simulink model "RS_DS_CM11_SimulinkRS"  (R2021b)
settings: Solver=ode1  StartTime=0.0  StopTime=Inf  FixedStep=0.001  RelTol=1e-3  EnableMultiTasking=on
PreLoadFcn:
  | if ~length(which('cmcmd')), cmenv; end
PostLoadFcn:
  | if any(exist('dsrtsu_mdlpostloadfcn', 'file') ~= 0), dsrtsu_mdlpostloadfcn('Execute', bdroot); end
InitFcn:
  | , if any(exist('rtifpga_mdlclblib', 'file') ~= 0), rtifpga_mdlclblib('Init', bdroot); end,
  | , if any(exist('dsmpb_private', 'file') ~= 0), dsmpb_private('dsmpb_mdlclblib', 'Init', bdroot); end,
  | runRS_SimulinkRS
values from neighbouring files (symbols this model uses):
  RealSimPara = struct    [runRS_SimulinkRS.m]    (also in runRS_noSimulinkRS.m)
libraries: CarMaker4SL x26, simulink x8, dsmpblib x7
(part 1 of 3)
PreSaveFcn:
  | , if any(exist('dsmpb_private', 'file') ~= 0), dsmpb_private('dsmpb_mdlclblib', 'PreSave', bdroot); end,
CloseFcn:
  | , if any(exist('dsmpb_private', 'file') ~= 0), dsmpb_private('dsmpb_mdlclblib', 'Close', bdroot); end,
settings Model: DSMPB_ID_DATA={'3029',struct('BlockId','959bbced-12c1-4767-83a1-89929a5713b7','SignalIds',{{'2dfba762-4a5d-4fb2-87c1-b3b2aa88a040'}}),'3030',struct('BlockId','c64a001f-194b-4229-bcb5-f85e1cedc51d','SignalIds',{{'b08fdf9a-de67-414c-8e8c-71615b990809'}}),'3031',struct('BlockId','a9d3bfec-9c38-4599-8c4c-82c07529655a','SignalIds',{{'89e99f5d-9eaf-4b55-ad87-136358e30858','260a6fdd-0a39-4666-a4ad-b2eb1261597d'}}),'3032',struct('BlockId','5c03b8fd-28bb-4541-b179-8665d7eb2a0a','SignalIds',{{'517e5a36-3f43-4f7c-bb45-a47e2302358f','00b36bbc-8fea-4739-bdae-9e60071a5ae6','c6bc667d-2809-40ad-8f52-15d7a7d0c444','b5810d90-0e08-4e08-a893-fc1e5645df05'}}),'3033',struct('BlockId','a9f3426c-e708-4ce6-abaa-842916ca8f03','SignalIds',{{'50966301-89aa-49cd-9e83-22a02fa0d1d9'}}),'3034',struct('BlockId','c86d215d-d6c6-481a-aa0d-d548a059715d','SignalIds',{{'abefa9c2-5971-43e2-92ea-8b98002a54ba','cddb9d5a-43dc-4246-b7b3-04f9827e0c24'}}),'3035',struct('BlockId','41a219ac-5dcc-4ef2-a113-31c003cb4a29','SignalIds',{{'3a4e41e0-0059-4009-8606-30e05f8817b4'}})}  RTICANMMDATA=struct('GeneralSetupData',struct('modelroot','C:\CM_Projects\RealSimCm11Prj\src_cm4sl','generalsettings',struct('filesettings',struct('destfolder',struct('Name','RTICANMM_FILES','Check',1),'buildfolder',struct('Name','.','Check',1),'AbsDestfolder',struct('Name','C:\CM_Projects\RealSimCm11Prj\src_cm4sl\RTICANMM_FILES'),'AbsBuildfolder',struct('Name','C:\CM_Projects\RealSimCm11Prj\src_cm4sl'))),'options',struct('addpaths',1,'rmpaths',1,'addtrcexclusion',true,'cannavigator',struct('checkmonitoring',0),'show_usrtrc',0,'use_usrtrc',0),'advanced',struct('options',ones(1,100)),'MPSetup',{{}},'RTI',struct('Type','DSRT','Ver','4.6','Date','02-Nov-2021'),'modelname','RS_DS_CM11_SimulinkRS','block','RS_DS_CM11_SimulinkRS'))  DSRTSU_INTERNAL_RTIFPGA=170  DSRTSU_INTERNAL_RTISTBM_VER=1.4.3  Creator=fh  LastModifiedBy=y0n
settings SolverCC: AlgebraicLoopSolver=TrustRegion
settings DataIOCC: LimitDataPoints=on  SaveFormat=Array  SignalLoggingSaveFormat=ModelDataLogs  ReturnWorkspaceOutputs=off  SignalLoggingName=sigsOut
settings OptimizationCC: BlockReduction=off  BooleanDataType=off  ConditionallyExecuteInputs=off  OptimizeBlockIOStorage=off  BufferReuse=off  GlobalBufferReuse=off  ExpressionFolding=off  ExpressionDepthLimit=2147483647  LocalBlockOutputs=off  InitFltsAndDblsToZero=on  OptimizeDataStoreBuffers=off  BusAssignmentInplaceUpdate=off
settings DebuggingCC: SaveWithParameterizedLinksMsg=none  UnderspecifiedInitializationDetection=Classic  MergeDetectMultiDrivingBlocksExec=none  SignalResolutionControl=TryResolveAllWithWarning  MultiTaskDSMMsg=warning  MultiTaskCondExecSysMsg=none  TasksWithSamePriorityMsg=none  FcnCallInpInsideContextMsg=warning  StateNameClashWarn=warning  SFUnexpectedBacktrackingDiag=warning  SFNoUnconditionalDefaultTransitionDiag=warning  SFMachineParentedDataDiag=warning  ArithmeticOperatorsInVariantConditions=warning
settings HardwareCC: ProdBitPerPointer=32  ProdBitPerSizeT=32  ProdBitPerPtrDiffT=32  ProdLargestAtomicInteger=Integer  ProdWordSize=32  ProdHWDeviceType=Custom Processor->Custom
settings ModelReferenceCC: PropagateSignalLabelsOutOfModel=off
settings SFSimCC: SimUseLocalCustomCode=off  MATLABDynamicMemAlloc=off  CustomCodeUndefinedFunction=UseInterfaceOnly
settings RTWCC: Description=dSPACE Run-Time Target (for VEOS on Windows and ConfigurationDesk)  SystemTargetFile=dsrt.tlc  GenCodeOnly=on  MakeCommand=make_dsrt  TemplateMakefile=dsrt_default_tmf  RTWVerbose=off  RTWUseLocalCustomCode=off
settings CodeAppCC: MaxIdLength=63  StateflowObjectComments=on
settings STFCustomTargetCC: ParMdlRefBuildCompliant=on  GRTInterface=off  SystemTargetFile=dsrt.tlc
settings GRTTargetCC: TargetLangStandard=C89/C90 (ANSI)  CompOptLevelCompliant=off  ConcurrentExecutionCompliant=off  CombineOutputUpdateFcns=off  MatFileLogging=off  CPPClassGenCompliant=off  UseToolchainInfoCompliant=off
settings ConfigComp: CovMetricSettings=dw  CovSaveCumulativeToWorkspaceVar=on  CovSaveSingleToWorkspaceVar=on  CovExternalEMLEnable=off

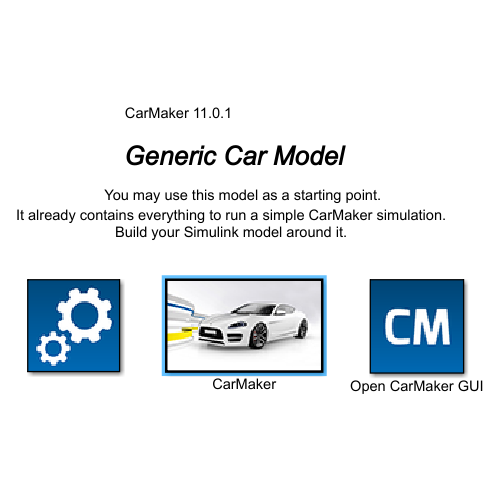
[thumbnail: Simulink's stored preview of the top-level diagram]
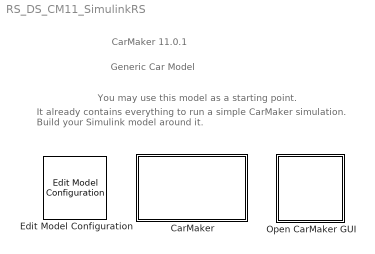
== system RS_DS_CM11_SimulinkRS ==
  note: Generic Car Model
  note: You may use this model as a starting point.
  note: It already contains everything to run a simple CarMaker simulation.
      | Build your Simulink model around it.
  note: CarMaker 11.0.1
  CarMaker : Subsystem  TreatAsAtomicUnit=on
      mask Display: image(imread('CarMakerSys.png'));
  Edit Model Configuration : CarMaker4SL/Edit Model Configuration  SFunctionModules=''
  Open CarMaker GUI : Subsystem  LoadFcn=if ~length(which('cmself')), cmenv; end
      settings: OpenFcn=cmblockmagic('gui_fix_display'); CM_HIL
      mask Display: image(imread('CarMakerGUI.png'));

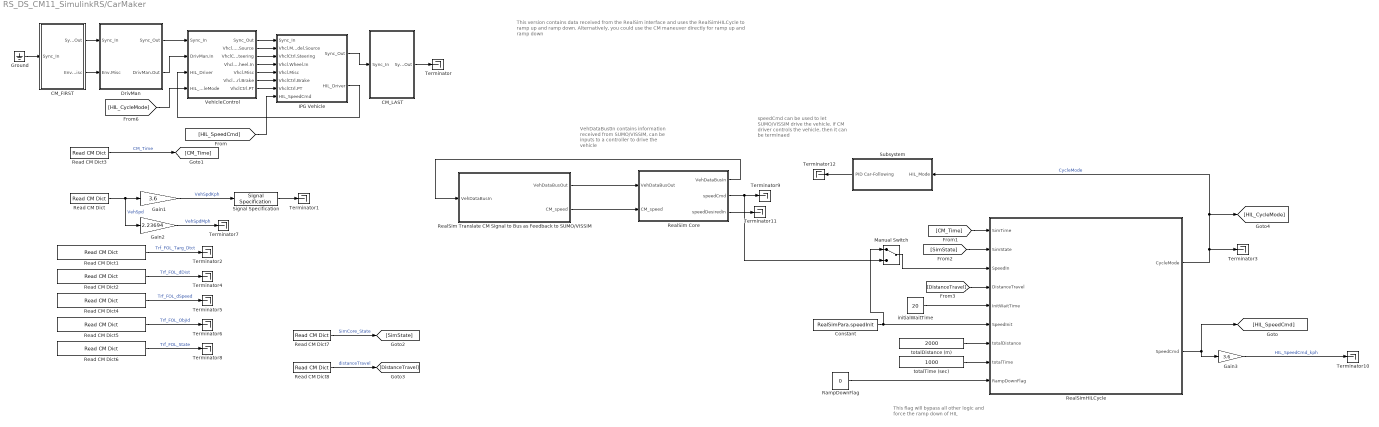
== system RS_DS_CM11_SimulinkRS/CarMaker ==
  note: This version contains data received from the RealSim interface and uses the RealSimHILCycle to ramp up and ramp down.
      |
      | Alternatively, you could use the CM maneuver directly for ramp up and ramp down
  note: speedCmd can be used to let SUMO/VISSIM drive the vehicle. if CM driver controls the vehicle, then it can be terminaed
  note: VehDataBustIn contains information received from SUMO/VISSIM, can be inputs to a controller to drive the vehicle
  note: This flag will bypass all other logic and force the ramp down of HIL
  CM_FIRST : Subsystem
  CM_LAST : Subsystem
  Constant : Constant  Value=RealSimPara.speedInit
  DrivMan : Subsystem
  Gain1 : Gain  Gain=3.6
  Gain2 : Gain  Gain=2.23694
  Gain3 : Gain  Gain=3.6
  Ground : Ground
  IPG Vehicle : Subsystem
  Manual Switch : ManualSwitch
  RampDownFlag : Constant  Value=0
  Read CM Dict : CarMaker4SL/Read CM Dict  xname=Car.v  xsync=off  xstime=Continuous
  Read CM Dict1 : CarMaker4SL/Read CM Dict  xname=Driver.ReCon.Trf_FOL.Targ_Dtct  xsync=off  xstime=Continuous
  Read CM Dict2 : CarMaker4SL/Read CM Dict  xname=Driver.ReCon.Trf_FOL.dDist  xsync=off  xstime=Continuous
  Read CM Dict3 : CarMaker4SL/Read CM Dict  xname=Time  xsync=off  xstime=Continuous
  Read CM Dict4 : CarMaker4SL/Read CM Dict  xname=Driver.ReCon.Trf_FOL.dSpeed  xsync=off  xstime=Continuous
  Read CM Dict5 : CarMaker4SL/Read CM Dict  xname=Driver.ReCon.Trf_FOL.ObjId  xsync=off  xstime=Continuous
  Read CM Dict6 : CarMaker4SL/Read CM Dict  xname=Driver.ReCon.Trf_FOL.State  xsync=off  xstime=Continuous
  Read CM Dict7 : CarMaker4SL/Read CM Dict  xname=SC.State  xsync=off  xstime=Continuous
  Read CM Dict8 : CarMaker4SL/Read CM Dict  xname=Vhcl.Distance  xsync=off  xstime=Continuous
  RealSim Core : Subsystem
  RealSim Translate CM Signal to Bus as Feedback to SUMO/VISSIM : Subsystem
  RealSimHILCycle : Stateflow chart  TreatAsAtomicUnit=on
  Signal Specification : SignalSpecification  Unit=km/h
  Subsystem : Subsystem
  Terminator{,1..12} (13 alike) : Terminator
  VehicleControl : Subsystem
  initialWaitTime : Constant  Value=20
  totalDistance (m) : Constant  Value=2000
  totalTime (sec) : Constant  Value=1000
  wires:
  DrivMan/2(DrivMan.Out) -> VehicleControl/2(DrivMan.In)
  DrivMan/1(Sync_Out) -> VehicleControl/1(Sync_In)
  CM_FIRST/2(Env.Misc) -> DrivMan/2(Env.Misc)
  CM_FIRST/1(Sync_Out) -> DrivMan/1(Sync_In)
  CM_LAST/1(Sync_Out) -> Terminator/1
  Ground/1 -> CM_FIRST/1(Sync_In)
  IPG Vehicle/1(Sync_Out) -> CM_LAST/1(Sync_In)
  VehicleControl/1(Sync_Out) -> IPG Vehicle/1(Sync_In)
  VehicleControl/3(VhclCtrl.Steering) -> IPG Vehicle/3(VhclCtrl.Steering)
  VehicleControl/4(Vhcl.Wheel.In) -> IPG Vehicle/4(Vhcl.Wheel.In)
  VehicleControl/5(Vhcl.Misc) -> IPG Vehicle/5(Vhcl.Misc)
  VehicleControl/6(VhclCtrl.Brake) -> IPG Vehicle/6(VhclCtrl.Brake)
  VehicleControl/7(VhclCtrl.PT) -> IPG Vehicle/7(VhclCtrl.PT)
  VehicleControl/2(Vhcl.Model.Source) -> IPG Vehicle/2(Vhcl.Model.Source)
  Read CM Dict3/1 -> [CM_Time]  "CM_Time"
  Read CM Dict/1 -> Gain2/1, Gain1/1  "VehSpd"
  Gain2/1 -> Terminator7/1  "VehSpdMph"
  Gain1/1 -> Signal Specification/1  "VehSpdKph"
  Signal Specification/1 -> Terminator1/1
  Read CM Dict1/1 -> Terminator2/1  "Trf_FOL_Targ_Dtct"
  Read CM Dict2/1 -> Terminator4/1  "Trf_FOL_dDist"
  Read CM Dict4/1 -> Terminator5/1  "Trf_FOL_dSpeed"
  Read CM Dict5/1 -> Terminator6/1  "Trf_FOL_ObjId"
  Read CM Dict6/1 -> Terminator8/1  "Trf_FOL_State"
  RealSim Core/2(speedCmd) -> Terminator9/1, Manual Switch/2
  RealSim Translate CM Signal to Bus as Feedback to SUMO/VISSIM/2(CM_speed) -> RealSim Core/2(CM_speed)
  RealSim Core/1(VehDataBusIn) -> RealSim Translate CM Signal to Bus as Feedback to SUMO/VISSIM/1(VehDataBusIn)
  RealSim Translate CM Signal to Bus as Feedback to SUMO/VISSIM/1(VehDataBusOut) -> RealSim Core/1(VehDataBusOut)
  Read CM Dict7/1 -> [SimState]  "SimCore_State"
  IPG Vehicle/2(HIL_Driver) -> VehicleControl/3(HIL_Driver)
  RealSim Core/3(speedDesiredIn) -> Terminator11/1
  [HIL_SpeedCmd] -> IPG Vehicle/8(HIL_SpeedCmd)
  Read CM Dict8/1 -> [DistanceTravel]  "distanceTravel"
  [SimState] -> RealSimHILCycle/2(SimState)
  Constant/1 -> RealSimHILCycle/6(SpeedInit), Manual Switch/1
  totalDistance (m)/1 -> RealSimHILCycle/7(totalDistance)
  [DistanceTravel] -> RealSimHILCycle/4(DistanceTravel)
  RealSimHILCycle/2(SpeedCmd) -> [HIL_SpeedCmd], Gain3/1
  Subsystem/1(PID Car-Following) -> Terminator12/1
  initialWaitTime/1 -> RealSimHILCycle/5(InitWaitTime)
  [CM_Time] -> RealSimHILCycle/1(SimTime)
  RealSimHILCycle/1(CycleMode) -> [HIL_CycleMode], Subsystem/1(HIL_Mode), Terminator3/1  "CycleMode"
  totalTime (sec)/1 -> RealSimHILCycle/8(totalTime)
  Manual Switch/1 -> RealSimHILCycle/3(SpeedIn)
  Gain3/1 -> Terminator10/1  "HIL_SpeedCmd_kph"
  RampDownFlag/1 -> RealSimHILCycle/9(RampDownFlag)
  [HIL_CycleMode] -> VehicleControl/4(HIL_CycleMode)

== system RS_DS_CM11_SimulinkRS/Open CarMaker GUI ==
  S-Function : S-Function  FunctionName=cm_gui  SFunctionDeploymentMode=off  EnableBusSupport=off

== system RS_DS_CM11_SimulinkRS/CarMaker/CM_FIRST ==
  Sync_In : Inport
  BusCreator1 : BusCreator  Inputs=8
  BusCreator2 : BusCreator  Inputs=6
  Demux1 : Demux  Outputs=14
      settings: DisplayOption=none
  Environment : S-Function  FunctionName=CM_Sfun  Parameters='Environment'  SFunctionDeploymentMode=off  EnableBusSupport=off
  IoIn : S-Function  FunctionName=CM_Sfun  Parameters='IoIn'  SFunctionDeploymentMode=off  EnableBusSupport=off
  Terminator : Terminator
  Sync_Out : Outport  VectorParamsAs1DForOutWhenUnconnected=off
  Env.Misc : Outport  Port=2  VectorParamsAs1DForOutWhenUnconnected=off
  wires:
  BusCreator2/1 -> Terminator/1  "IF Environment (in)"
  BusCreator1/1 -> Env.Misc/1
  Demux1/14 -> BusCreator2/6  "Env sRoad"
  Demux1/13 -> BusCreator2/5  "Env PoI_GCS Elev"
  Demux1/12 -> BusCreator2/4  "Env PoI_GCS Lat"
  Demux1/11 -> BusCreator2/3  "Env PoI_GCS Long"
  Demux1/10 -> BusCreator2/2  "Env Time"
  Demux1/9 -> BusCreator2/1  "Env yDay"
  Demux1/8 -> BusCreator1/8  "Env WindVel_tot z"
  Demux1/7 -> BusCreator1/7  "Env WindVel_tot y"
  Demux1/6 -> BusCreator1/6  "Env WindVel_tot x"
  Demux1/5 -> BusCreator1/5  "Env SolarRadiation"
  Demux1/4 -> BusCreator1/4  "Env AirHumidity"
  Demux1/3 -> BusCreator1/3  "Env AirPressure"
  Demux1/2 -> BusCreator1/2  "Env AirDensity"
  Demux1/1 -> BusCreator1/1  "Env Temperature"
  Environment/2 -> Demux1/1
  Environment/1 -> Sync_Out/1
  IoIn/1 -> Environment/1
  Sync_In/1 -> IoIn/1

== system RS_DS_CM11_SimulinkRS/CarMaker/CM_LAST ==
  Sync_In : Inport
  CM_User : S-Function  FunctionName=CM_Sfun  Parameters='CM_User'  SFunctionDeploymentMode=off  EnableBusSupport=off
  IoOut : S-Function  FunctionName=CM_Sfun  Parameters='IoOut'  SFunctionDeploymentMode=off  EnableBusSupport=off
  Sync_Out : Outport  VectorParamsAs1DForOutWhenUnconnected=off
  wires:
  IoOut/1 -> Sync_Out/1
  CM_User/1 -> IoOut/1
  Sync_In/1 -> CM_User/1

== system RS_DS_CM11_SimulinkRS/CarMaker/DrivMan ==
  note: There's rarely a reason to override DrivMan signals.
      | Use the VehicleControl interface for this purpose.
  Sync_In : Inport
  Env.Misc : Inport  Port=2
  BusCreator : BusCreator  Inputs=17
  Demux : Demux  Outputs=17
      settings: DisplayOption=none
  DrivMan : S-Function  FunctionName=CM_Sfun  Parameters='DrivMan'  SFunctionDeploymentMode=off  EnableBusSupport=off
  Sync_Out : Outport  VectorParamsAs1DForOutWhenUnconnected=off
  DrivMan.Out : Outport  Port=2  VectorParamsAs1DForOutWhenUnconnected=off
  wires:
  Demux/17 -> BusCreator/17  "DrivMan Steering Trq"
  Demux/16 -> BusCreator/16  "DrivMan Steering AngAcc"
  Demux/15 -> BusCreator/15  "DrivMan Steering AngVel"
  Demux/14 -> BusCreator/14  "DrivMan Steering Ang"
  Demux/13 -> BusCreator/13  "DrivMan Gas"
  Demux/12 -> BusCreator/12  "DrivMan Clutch"
  Demux/11 -> BusCreator/11  "DrivMan BrakePark"
  Demux/10 -> BusCreator/10  "DrivMan Brake"
  Demux/9 -> BusCreator/9  "DrivMan GearNo"
  Demux/8 -> BusCreator/8  "DrivMan SelectorCtrl"
  Demux/7 -> BusCreator/7  "DrivMan UserSignal4"
  Demux/6 -> BusCreator/6  "DrivMan UserSignal3"
  Demux/5 -> BusCreator/5  "DrivMan UserSignal2"
  Demux/4 -> BusCreator/4  "DrivMan UserSignal1"
  Demux/3 -> BusCreator/3  "DrivMan UserSignal0"
  Demux/2 -> BusCreator/2  "DrivMan Key"
  Demux/1 -> BusCreator/1  "DrivMan SST"
  Env.Misc/1 -> DrivMan/2
  Sync_In/1 -> DrivMan/1
  DrivMan/1 -> Sync_Out/1
  BusCreator/1 -> DrivMan.Out/1
  DrivMan/2 -> Demux/1

== system RS_DS_CM11_SimulinkRS/CarMaker/IPG Vehicle ==
  Sync_In : Inport
  Vhcl.Model.Source : Inport  Port=2
  VhclCtrl.Steering : Inport  Port=3
  Vhcl.Wheel.In : Inport  Port=4
  Vhcl.Misc : Inport  Port=5
  VhclCtrl.Brake : Inport  Port=6
  VhclCtrl.PT : Inport  Port=7
  HIL_SpeedCmd : Inport  Port=8
  Actuation and Outputs : Subsystem
  Brake : Subsystem
  CarAndTrailer : Subsystem
  Driver and Drive Cycle : Subsystem  TreatAsAtomicUnit=on
  Gain1 : Gain  Gain=3.6
  Gain2 : Gain  Gain=2.23694
  Gain3 : Gain  Gain=3.6
  PowerTrain : Subsystem
  Read CM Dict : CarMaker4SL/Read CM Dict  xname=Car.v  xsync=off  xstime=Continuous
  Signal Specification : SignalSpecification  Unit=km/h
  Stop Simulation : Stop
  Terminator : Terminator
  Terminator7 : Terminator
  VehicleSource_BuiltIn : simulink/Logic and Bit Operations/Compare To Constant  relop=~=  const=1  OutDataTypeStr=boolean  ZeroCross=off
  Sync_Out : Outport  VectorParamsAs1DForOutWhenUnconnected=off
  HIL_Driver : Outport  Port=2
  wires:
  VhclCtrl.PT/1 -> [VhclCtrl_PT], PowerTrain/3(VhclCtrl.PT)
  Brake/1(Sync_Out) -> PowerTrain/1(Sync_In)
  CarAndTrailer/1(Sync_Out) -> Brake/1(Sync_In)
  CarAndTrailer/2(Brake.IF.In) -> Brake/2(Brake.IF.In)
  VhclCtrl.Brake/1 -> Brake/3(VhclCtrl.Brake)
  PowerTrain/1(Sync_Out) -> Sync_Out/1
  Vhcl.Misc/1 -> CarAndTrailer/4(Vhcl.Misc)
  Vhcl.Wheel.In/1 -> CarAndTrailer/3(Vhcl.Wheel.In)
  VhclCtrl.Steering/1 -> CarAndTrailer/2(VhclCtrl.Steering)
  Sync_In/1 -> CarAndTrailer/1(Sync_In)
  Vhcl.Model.Source/1 -> VehicleSource_BuiltIn/1
  VehicleSource_BuiltIn/1 -> Stop Simulation/1
  Brake/2(Vhcl.Wheel.PT) -> PowerTrain/2(Vhcl.Wheel.PT)
  [VhclCtrl_PT] -> Actuation and Outputs/2(CM Driver Commands)
  Gain1/1 -> Signal Specification/1  "VehSpdKph"
  Driver and Drive Cycle/1(DriverBus) -> Actuation and Outputs/1(HIL Driver Commands)
  Actuation and Outputs/2(HIL_Driver) -> HIL_Driver/1
  Signal Specification/1 -> Driver and Drive Cycle/1(Veh speed feedback [kph]), [VehSpdKph]
  Read CM Dict/1 -> [VehSpd], Gain2/1, Gain1/1  "VehSpd"
  Gain2/1 -> Terminator7/1  "VehSpdMph"
  Actuation and Outputs/1(BrakeSwitch) -> Terminator/1
  HIL_SpeedCmd/1 -> Gain3/1
  Gain3/1 -> Driver and Drive Cycle/2(HIL Veh speed Cmd [kph])  "VehSpdKph"

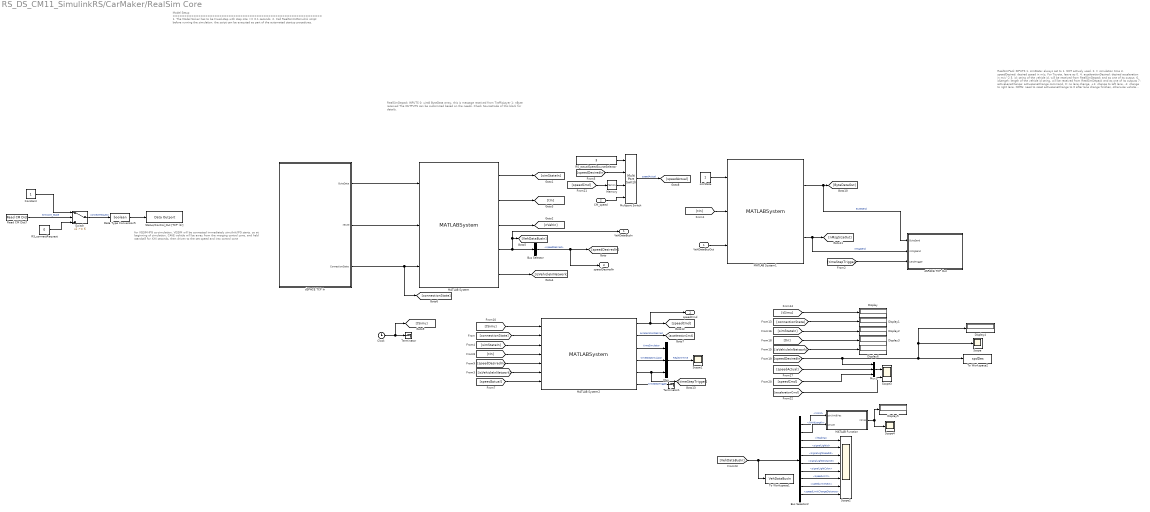
== system RS_DS_CM11_SimulinkRS/CarMaker/RealSim Core ==
  note: Model Setup
      | ================================================================
      | 1. The Model Solver has to be Fixed-step with step size <= 0.1 seconds.
      | 2. Call RealSimInitSimulink script before running the simulation. the script can be executed as part of the automated startup procedures.
  note: RealSimDepack
      | INPUTS
      | 0: uint8 ByteData array, this is message received from TrafficLayer
      | 1: nByte received
      |
      | The OUTPUTS can be customized based on the needs. Check SourceCode of this block for details.
  note: RealSimPack
      | INPUTS
      | 1. simState: always set to 1. NOT actively used.
      | 2. t: simulation time
      | 3. speedDesired: desired speed in m/s, For Toyota, leave as 0.
      | 4. accelerationDesired: desired acceleration in m/s^2
      | 5. id: string of the vehicle id, will be received from RealSimDepack and as one of its output.
      | 6. idLength: length of the vehicle id string, will be received from RealSimDepack and as one of its outputs
      | 7: activeLaneChange: activeLaneChange command, 0: no lane change, +1: change to left lane, -1: change to right lane. NOTE: need to reset activeLaneChange to 0 after lane change finishes, otherwise vehicle will keep making lane change. Will receive 0 activeLaneChangeFdbk from RealSimDepack when lane change finishes.
      |
      | NOTE 1: Currently, only speedDesired and/or accelerationDesired can be sent to VISSIM/SUMO. The data format receive and send are the same so other mesage fields of the send data are irrelevant and can be set to empty or zero.
      |
      | NOTE 2: if select both speedDesired and accelerationDesired
      | in config.yaml, then only accelerationDesired will be used
      | to control vehicles in TrafficSimulator. if only one of
      | speedDesired and accelerationDesired selected in
      | config.yaml, then the one selected will be used for
      | control, the other input can be leave as 0.
      |
      | NOTE 3: for VISSIM, speedDesired or accelerationDesired will be the control command 0.2 seconds in the future.
      |
      | OUTPUTS
      | 1.ByteData: bytes vector that will be sent to TrafficSimualtor
      | 2.nMsgSize: size of bytes to be sent
  note: for VISSIM-IPG co-simulation, VISSIM will be connected immediately simulink/IPG starts. so at beginning of simulation, CAVE vehicle will be away from the merging control zone, and held standstill for XXX seconds, then driven to the set speed and into control zone
  VehDataBusOut : Inport
  CM_speed : Inport  Port=2
  Bus Selector : BusSelector  OutputSignals=speedDesired
  Bus Selector2 : BusSelector  OutputSignals=linkId,linkIdLength,heading,signalLightId,signalLightHeadId,signalLightDistance,signalLightColor,speedLimit,speedLimitNext,speedLimitChangeDistance
  Clock : Clock
  Constant : Constant
  Data Type Conversion5 : DataTypeConversion  OutDataTypeStr=boolean
  Display{,1..6} (7 alike) : Display
  MATLAB Function : MATLAB Function  TreatAsAtomicUnit=on
  MATLAB System : MATLABSystem  System=RealSimDepack  OutputBusName=VehDataBus  VehicleMessageFieldDefInputVec=VehicleMessageFieldDefInputVec  SimulateUsing=Code generation
      mask Type: RealSimDepack
      mask Display:
      | disp('RealSimDepack');
      | port_label('input',1,'ByteData');
      | port_label('input',2,'nByte');
      | port_label('input',3,'connectionState');
      | port_label('output',1,'simState');
      | port_label('output',2,'t');
      | port_label('output',3,'nVeh');
      | port_label('output',4,'VehDataBus');
      | port_label('output',5,'isVehicleInNetwork');
  MATLAB System1 : MATLABSystem  System=RealSimPack  VehicleMessageFieldDefInputVec=VehicleMessageFieldDefInputVec  SimulateUsing=Code generation
      mask Type: RealSimPack
      mask Display:
      | disp('RealSimPack');
      | port_label('input',1,'simState');
      | port_label('input',2,'t');
      | port_label('input',3,'VehDataBus');
      | port_label('output',1,'ByteData');
      | port_label('output',2,'nMsgSize');
  MATLAB System2 : MATLABSystem  System=RealSimInterpSpeed  initialSpeed=RealSimPara.speedInit  speedLookAheadHorizon=RealSimPara.tLookahead  speedUpperBound=30  smoothWindow=RealSimPara.smoothWindow  SimulateUsing=Code generation
      mask Type: RealSimInterpSpeed
      mask Display:
      | disp('RealSimInterpSpeed');
      | port_label('input',1,'simulationTime');
      | port_label('input',2,'connectionState');
      | port_label('input',3,'simState');
      | port_label('input',4,'timeReceive');
      | port_label('input',5,'speedReceive');
      | port_label('input',6,'isVehicleInNetwork');
      | port_label('input',7,'speedActual');
      | port_label('output',1,'speedLookAhead');
      | port_label('output',2,'accelerationDesired');
      | port_label('output',3,'timeSimulator');
      | port_label('output',4,'timeStepSimulator');
      | port_label('output',5,'timeStepTrigger');
      | port_label('output',6,'RealSimDelay');
  Memory : Memory
  Multiport Switch : MultiPortSwitch
  Mux : Mux  Inputs=3
  Mux1 : Mux  Inputs=3
  RS_actualSpeedSourceSelector : Constant  Value=3
  RS_connectRequest : Constant  Value=0
  Read CM Dict7 : CarMaker4SL/Read CM Dict  xname=SC.State  xsync=off  xstime=Continuous
  Scope : Scope
  Scope1 : Scope
  Scope2 : Scope  NumInputPorts=8
  Scope3 : Scope  NumInputPorts=2
  Scope4 : Scope
  Status/Control_Out [TCP (1)] : dsmpblib/Data Outport  Priority=-10000
      settings: SourceProductName=dSPACE Model Interface Blockset
  Switch : Switch  Threshold=6
  Terminator : Terminator
  Terminator1 : Terminator
  To Workspace1 : ToWorkspace  VariableName=VehDataBusIn  SaveFormat=Timeseries  SampleTime=-1
  To Workspace2 : ToWorkspace  VariableName=spdDes  SaveFormat=Structure With Time  SampleTime=-1
  dSPACE TCP In : Subsystem
  dSPACE TCP Out : Subsystem
  simState : Constant
  VehDataBusIn : Outport
  speedCmd : Outport  Port=2
  speedDesiredIn : Outport  Port=3
  wires:
  [speedCmd] -> Memory/1
  Bus Selector/1 -> speedDesiredIn/1, [speedDesiredIn]  "<speedDesired>"
  MATLAB System/1 -> [simStateIn]
  Bus Selector2/9 -> Scope2/7  "<speedLimitNext>"
  [tSimu] -> MATLAB System2/1
  MATLAB System2/4 -> Mux/2  "timeStepSimulator"
  Bus Selector2/1 -> MATLAB Function/1(strUint8Vec)  "<linkId>"
  Bus Selector2/3 -> Scope2/1  "<heading>"
  [tIn] -> MATLAB System2/4
  Bus Selector2/10 -> Scope2/8  "<speedLimitChangeDistance>"
  CM_speed/1 -> Multiport Switch/4
  [speedDesiredIn] -> MATLAB System2/5
  [simStateIn] -> Display2/1
  MATLAB System/3 -> [nVehIn]
  [VehDataBusIn] -> To Workspace1/1, Bus Selector2/1
  [isVehicleInNetwork] -> Display6/1
  Bus Selector2/7 -> Scope2/5  "<signalLightColor>"
  simState/1 -> MATLAB System1/1
  MATLAB System/4 -> VehDataBusIn/1, [VehDataBusIn], Bus Selector/1
  [speedDesiredIn] -> Display4/1, Scope/1, To Workspace2/1, Mux1/1
  MATLAB System2/2 -> [accelerationCmd]  "accelerationDesired"
  [isVehicleInNetwork] -> MATLAB System2/6
  RS_actualSpeedSourceSelector/1 -> Multiport Switch/1
  VehDataBusOut/1 -> MATLAB System1/3
  [accelerationCmd] -> Scope3/2
  Mux/1 -> Scope1/1  "RealSimTime"
  [tIn] -> MATLAB System1/2
  Bus Selector2/2 -> MATLAB Function/2(strLen)  "<linkIdLength>"
  Bus Selector2/8 -> Scope2/6  "<speedLimit>"
  [connectionState] -> Display1/1
  MATLAB System2/5 -> [timeStepTrigger], Mux/3  "timeStepTrigger"
  MATLAB System/5 -> [isVehicleInNetwork]
  Bus Selector2/5 -> Scope2/3  "<signalLightHeadId>"
  Bus Selector2/6 -> Scope2/4  "<signalLightDistance>"
  MATLAB System2/6 -> Terminator1/1
  MATLAB System1/1 -> dSPACE TCP Out/1(ByteSend), [ByteDataOut]  "ByteSend"
  [tIn] -> Display3/1
  Multiport Switch/1 -> [speedActual]  "speedActual"
  [tSimu] -> Display/1
  [connectionState] -> MATLAB System2/2
  [speedCmd] -> Mux1/3
  [speedActual] -> MATLAB System2/7
  [simStateIn] -> MATLAB System2/3
  MATLAB System2/1 -> speedCmd/1, [speedCmd]
  Mux1/1 -> Scope3/1
  MATLAB Function/1(intVal) -> Scope4/1, Display5/1
  MATLAB System1/2 -> dSPACE TCP Out/2(nMsgSend), [nMsgSizeOut]  "nMsgSend"
  Bus Selector2/4 -> Scope2/2  "<signalLightId>"
  MATLAB System2/3 -> Mux/1  "timeSimulator"
  [speedDesiredIn] -> Multiport Switch/2
  [speedActual] -> Mux1/2
  MATLAB System/2 -> [tIn]
  [timeStepTrigger] -> dSPACE TCP Out/3(sendTrigger)
  dSPACE TCP In/3(ConnectionState) -> [connectionState], MATLAB System/3
  dSPACE TCP In/1(ByteData) -> MATLAB System/1
  dSPACE TCP In/2(nByte) -> MATLAB System/2
  Data Type Conversion5/1 -> Status/Control_Out [TCP (1)]/1
  Switch/1 -> Data Type Conversion5/1  "connectRequest"
  Memory/1 -> Multiport Switch/3
  Clock/1 -> Terminator/1, [tSimu]
  RS_connectRequest/1 -> Switch/3
  Read CM Dict7/1 -> Switch/2  "SimCore_State"
  Constant/1 -> Switch/1

== system RS_DS_CM11_SimulinkRS/CarMaker/RealSim Translate CM Signal to Bus as Feedback to SUMO//VISSIM ==
  VehDataBusIn : Inport
  Constant : Constant  Value=[255,0,0,255]
  Constant3 : Constant  Value=0
  MATLAB Function : MATLAB Function  TreatAsAtomicUnit=on
  Read CM Dict : CarMaker4SL/Read CM Dict  xname=Vhcl.Fr1.x  xsync=off  xstime=Continuous
  Read CM Dict1 : CarMaker4SL/Read CM Dict  xname=Vhcl.PoI.x  xsync=off  xstime=Continuous
  Read CM Dict2 : CarMaker4SL/Read CM Dict  xname=Vhcl.v  xsync=off  xstime=Continuous
  Read CM Dict3 : CarMaker4SL/Read CM Dict  xname=Vhcl.Yaw  xsync=off  xstime=Continuous
  Read CM Dict4 : CarMaker4SL/Read CM Dict  xname=Vhcl.Fr1.y  xsync=off  xstime=Continuous
  Read CM Dict5 : CarMaker4SL/Read CM Dict  xname=Vhcl.Fr1.z  xsync=off  xstime=Continuous
  Read CM Dict6 : CarMaker4SL/Read CM Dict  xname=Vhcl.PoI.y  xsync=off  xstime=Continuous
  Read CM Dict7 : CarMaker4SL/Read CM Dict  xname=Vhcl.PoI.z  xsync=off  xstime=Continuous
  RealSim CreatBus : Subsystem
  VehDataBusOut : Outport
  CM_speed : Outport  Port=2
  wires:
  Read CM Dict6/1 -> MATLAB Function/2(CM_POI_Y)
  MATLAB Function/6(speedDesired) -> RealSim CreatBus/7(speedDesired)
  MATLAB Function/4(heading) -> RealSim CreatBus/5(heading)
  Read CM Dict2/1 -> CM_speed/1, MATLAB Function/9(CM_speed)
  Read CM Dict4/1 -> MATLAB Function/5(CM_Fr1_Y)
  MATLAB Function/2(positionY) -> RealSim CreatBus/3(positionY)
  MATLAB Function/1(positionX) -> RealSim CreatBus/2(positionX)
  Read CM Dict/1 -> MATLAB Function/4(CM_Fr1_X)
  MATLAB Function/3(positionZ) -> RealSim CreatBus/4(positionZ)
  Read CM Dict7/1 -> MATLAB Function/3(CM_POI_Z)
  MATLAB Function/5(color) -> RealSim CreatBus/6(color)
  Constant/1 -> MATLAB Function/8(color_rgba)
  Read CM Dict5/1 -> MATLAB Function/6(CM_Fr1_Z)
  Read CM Dict1/1 -> MATLAB Function/1(CM_POI_X)
  Read CM Dict3/1 -> MATLAB Function/7(CM_yaw)
  VehDataBusIn/1 -> RealSim CreatBus/1(In)
  RealSim CreatBus/1(Out) -> VehDataBusOut/1

== system RS_DS_CM11_SimulinkRS/CarMaker/Subsystem ==
  HIL_Mode : Inport
  Add2 : Sum
  Add3 : Sum
  Constant1 : Constant  Value=10
  Divide : Product  Inputs=**
  PID Speed Driver : Subsystem
  Read CM Dict10 : CarMaker4SL/Read CM Dict  xname=Driver.ReCon.Trf_FOL.Targ_Dtct  xsync=off  xstime=Continuous
  Read CM Dict11 : CarMaker4SL/Read CM Dict  xname=Car.v  xsync=off  xstime=Continuous
  Read CM Dict12 : CarMaker4SL/Read CM Dict  xname=Driver.ReCon.Trf_FOL.dDist  xsync=off  xstime=Continuous
  Read CM Dict9 : CarMaker4SL/Read CM Dict  xname=Driver.ReCon.Trf_FOL.dSpeed  xsync=off  xstime=Continuous
  Switch : Switch  Criteria=u2 > Threshold
  free speed : Constant  Value=RealSimPara.speedInit
  headway (s) : Constant  Value=4
  PID Car-Following : Outport
  wires:
  Divide/1 -> Add3/2
  Add2/1 -> Switch/1, [precedingSpeed]  "Trf_Prec_Speed"
  Switch/1 -> PID Speed Driver/2(RefSpd)  "RefSpd"
  [precedingSpeed] -> Divide/1
  Read CM Dict11/1 -> PID Speed Driver/3(VehicleSpeed), Add2/1
  Read CM Dict9/1 -> Add2/2  "Trf_FOL_dSpeed"
  Read CM Dict12/1 -> PID Speed Driver/5(FollowDistance)  "Trf_FOL_dDist"
  Read CM Dict10/1 -> Switch/2  "Trf_FOL_Targ_Dtct"
  HIL_Mode/1 -> PID Speed Driver/1(speedSourceSwitch)
  free speed/1 -> Switch/3  "freeSpeed"
  Add3/1 -> PID Speed Driver/4(RefFollowDist)  "followingDistanceDesired"
  Constant1/1 -> Add3/1  "dMin"
  headway (s)/1 -> Divide/2  "headway"
  PID Speed Driver/1(Drv_Speed_Cmd) -> PID Car-Following/1

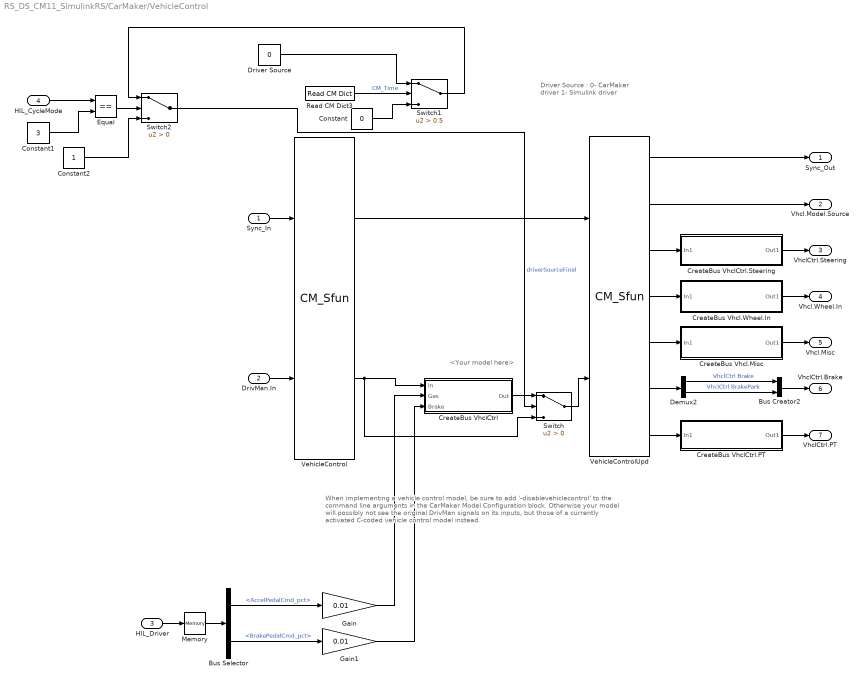
== system RS_DS_CM11_SimulinkRS/CarMaker/VehicleControl ==
  note: When implementing a vehicle control model,
      | be sure to add '-disablevehiclecontrol' to the command line arguments
      | in the CarMaker Model Configuration block.
      | Otherwise your model will possibly not see the original DrivMan signals
      | on its inputs, but those of a currently activated C-coded vehicle control model instead.
  note: <Your model here>
  note: Driver Source :
      | 0- CarMaker driver
      | 1- Simulink driver
  Sync_In : Inport
  DrivMan.In : Inport  Port=2
  HIL_Driver : Inport  Port=3
  HIL_CycleMode : Inport  Port=4
  Bus Creator2 : BusCreator  Inputs=2
  Bus Selector : BusSelector  OutputSignals=AccelPedalCmd_pct,BrakePedalCmd_pct
  Constant : Constant  Value=0
  Constant1 : Constant  Value=3
  Constant2 : Constant
  CreateBus Vhcl.Misc : Subsystem
  CreateBus Vhcl.Wheel.In : Subsystem
  CreateBus VhclCtrl : Subsystem
  CreateBus VhclCtrl.PT : Subsystem
  CreateBus VhclCtrl.Steering : Subsystem
  Demux2 : Demux  Outputs=2
      settings: DisplayOption=none
  Driver Source : Constant  Value=0
  Equal : RelationalOperator  Operator===  OutDataTypeStr=boolean  RndMeth=Simplest
  Gain : Gain  Gain=0.01
  Gain1 : Gain  Gain=0.01
  Memory : Memory  InheritSampleTime=on
  Read CM Dict3 : CarMaker4SL/Read CM Dict  xname=Time  xsync=off  xstime=Continuous
  Switch : Switch  Criteria=u2 > Threshold
  Switch1 : Switch  Criteria=u2 > Threshold  Threshold=0.5
  Switch2 : Switch  Criteria=u2 > Threshold
  VehicleControl : S-Function  FunctionName=CM_Sfun  Parameters='VehicleControl'  SFunctionDeploymentMode=off  EnableBusSupport=off
  VehicleControlUpd : S-Function  FunctionName=CM_Sfun  Parameters='VehicleControlUpd'  SFunctionDeploymentMode=off  EnableBusSupport=off
  Sync_Out : Outport
  Vhcl.Model.Source : Outport  Port=2
  VhclCtrl.Steering : Outport  Port=3
  Vhcl.Wheel.In : Outport  Port=4
  Vhcl.Misc : Outport  Port=5
  VhclCtrl.Brake : Outport  Port=6
  VhclCtrl.PT : Outport  Port=7
  wires:
  VehicleControlUpd/2 -> Vhcl.Model.Source/1
  VehicleControlUpd/4 -> CreateBus Vhcl.Wheel.In/1(In1)
  VehicleControlUpd/5 -> CreateBus Vhcl.Misc/1(In1)
  VehicleControlUpd/6 -> Demux2/1
  VehicleControlUpd/7 -> CreateBus VhclCtrl.PT/1(In1)
  VehicleControlUpd/3 -> CreateBus VhclCtrl.Steering/1(In1)
  CreateBus Vhcl.Misc/1(Out1) -> Vhcl.Misc/1
  CreateBus Vhcl.Wheel.In/1(Out1) -> Vhcl.Wheel.In/1
  DrivMan.In/1 -> VehicleControl/2
  VehicleControl/1 -> VehicleControlUpd/1
  Sync_In/1 -> VehicleControl/1
  CreateBus VhclCtrl.PT/1(Out1) -> VhclCtrl.PT/1
  Bus Creator2/1 -> VhclCtrl.Brake/1
  CreateBus VhclCtrl.Steering/1(Out1) -> VhclCtrl.Steering/1
  VehicleControlUpd/1 -> Sync_Out/1
  Demux2/2 -> Bus Creator2/2  "VhclCtrl BrakePark"
  Demux2/1 -> Bus Creator2/1  "VhclCtrl Brake"
  Bus Selector/1 -> Gain/1  "<AccelPedalCmd_pct>"
  HIL_Driver/1 -> Memory/1
  Bus Selector/2 -> Gain1/1  "<BrakePedalCmd_pct>"
  Memory/1 -> Bus Selector/1
  Gain/1 -> CreateBus VhclCtrl/2(Gas)
  VehicleControl/2 -> Switch/3, CreateBus VhclCtrl/1(In)
  Gain1/1 -> CreateBus VhclCtrl/3(Brake)
  CreateBus VhclCtrl/1(Out) -> Switch/1
  Switch/1 -> VehicleControlUpd/2
  Read CM Dict3/1 -> Switch1/2  "CM_Time"
  Driver Source/1 -> Switch1/1
  Constant/1 -> Switch1/3
  HIL_CycleMode/1 -> Equal/1
  Constant1/1 -> Equal/2
  Equal/1 -> Switch2/2
  Constant2/1 -> Switch2/3
  Switch1/1 -> Switch2/1
  Switch2/1 -> Switch/2  "driverSourceFinal"

== system RS_DS_CM11_SimulinkRS/CarMaker/IPG Vehicle/Actuation and Outputs ==
  note: Driver Commands are [0,100] for both pedal and brake
  HIL Driver Commands : Inport
  CM Driver Commands : Inport  Port=2
  APP : Constant  Value=0
  AR_limit : Saturate  UpperLimit=100  LowerLimit=0
  BR_command_0to100 : Constant  Value=0
  BR_limit : Saturate  UpperLimit=100  LowerLimit=0
  Bus Creator : BusCreator  Inputs=2
  Bus Selector : BusSelector  OutputSignals=VhclCtrl Gas
  Bus Selector1 : BusSelector  OutputSignals=AccelPedalCmd
  Bus Selector2 : BusSelector  OutputSignals=VhclCtrl Brake
  Bus Selector3 : BusSelector  OutputSignals=BrakePedalCmd
  Constant : Constant  Value=0
  Constant1 : Constant  Value=0
  Driver Control Selection : Constant  Value=2
  Gain1 : Gain  Gain=100
  Gain2 : Gain  Gain=100
  Min threshold for Brake switch : Constant  Value=0
  Multiport Switch1 : MultiPortSwitch  Inputs=4
  Multiport Switch2 : MultiPortSwitch  Inputs=4
  Relational Operator : RelationalOperator  Operator=>  OutDataTypeStr=boolean  RndMeth=Nearest
  BrakeSwitch : Outport  VectorParamsAs1DForOutWhenUnconnected=off
  HIL_Driver : Outport  Port=2
  wires:
  Multiport Switch1/1 -> AR_limit/1
  APP/1 -> Multiport Switch1/2
  Bus Selector1/1 -> Multiport Switch1/3  "<AccelPedalCmd>"
  Bus Selector/1 -> Gain2/1  "<VhclCtrl Gas>"
  Gain2/1 -> Multiport Switch1/4
  Multiport Switch2/1 -> BR_limit/1
  Gain1/1 -> Multiport Switch2/4
  HIL Driver Commands/1 -> Bus Selector3/1, Bus Selector1/1
  Bus Selector2/1 -> Gain1/1  "<VhclCtrl Brake>"
  Driver Control Selection/1 -> Multiport Switch1/1, Multiport Switch2/1
  BR_command_0to100/1 -> Multiport Switch2/2
  CM Driver Commands/1 -> Bus Selector2/1, Bus Selector/1
  Bus Selector3/1 -> Multiport Switch2/3  "<BrakePedalCmd>"
  Min threshold for Brake switch/1 -> Relational Operator/2
  Relational Operator/1 -> BrakeSwitch/1  "BrakeSwitch"
  Constant/1 -> Multiport Switch1/5
  Constant1/1 -> Multiport Switch2/5
  Bus Creator/1 -> HIL_Driver/1
  AR_limit/1 -> Bus Creator/1  "AccelPedalCmd_pct"
  BR_limit/1 -> Bus Creator/2, Relational Operator/1  "BrakePedalCmd_pct"

== system RS_DS_CM11_SimulinkRS/CarMaker/IPG Vehicle/Brake ==
  note: When replacing the entire braking system,
      | be sure to disable the IPG brake model by using the brake
      | model 'Model Manager off' in the vehicle GUI.
  note: <Your model here>
  Sync_In : Inport
  Brake.IF.In : Inport  Port=2
  VhclCtrl.Brake : Inport  Port=3
  Brake : S-Function  FunctionName=CM_Sfun  Parameters='Brake'  SFunctionDeploymentMode=off  EnableBusSupport=off
  BrakeUpd : S-Function  FunctionName=CM_Sfun  Parameters='BrakeUpd'  SFunctionDeploymentMode=off  EnableBusSupport=off
  BusCreator1 : BusCreator  Inputs=16
  CreateBus Vhcl.Wheel.PT : Subsystem
  Demux : Demux  Outputs=16
      settings: DisplayOption=none
  Sync_Out : Outport  VectorParamsAs1DForOutWhenUnconnected=off
  Vhcl.Wheel.PT : Outport  Port=2  VectorParamsAs1DForOutWhenUnconnected=off
  wires:
  Demux/16 -> BusCreator1/16  "Brake IF Trq_DriveSrc_trg d3"
  Demux/15 -> BusCreator1/15  "Brake IF Trq_DriveSrc_trg d2"
  Demux/14 -> BusCreator1/14  "Brake IF Trq_DriveSrc_trg d1"
  Demux/13 -> BusCreator1/13  "Brake IF Trq_DriveSrc_trg d0"
  Demux/12 -> BusCreator1/12  "Brake IF Trq_Reg_trg RR"
  Demux/11 -> BusCreator1/11  "Brake IF Trq_Reg_trg RL"
  Demux/10 -> BusCreator1/10  "Brake IF Trq_Reg_trg FR"
  Demux/9 -> BusCreator1/9  "Brake IF Trq_Reg_trg FL"
  Demux/8 -> BusCreator1/8  "Brake IF Trq_PB RR"
  Demux/7 -> BusCreator1/7  "Brake IF Trq_PB RL"
  Demux/6 -> BusCreator1/6  "Brake IF Trq_PB FR"
  Demux/5 -> BusCreator1/5  "Brake IF Trq_PB FL"
  Demux/4 -> BusCreator1/4  "Brake IF Trq_WB RR"
  Demux/3 -> BusCreator1/3  "Brake IF Trq_WB RL"
  Demux/2 -> BusCreator1/2  "Brake IF Trq_WB FR"
  Demux/1 -> BusCreator1/1  "Brake IF Trq_WB FL"
  Brake/2 -> Demux/1
  BusCreator1/1 -> BrakeUpd/2
  BrakeUpd/1 -> Sync_Out/1
  Brake/1 -> BrakeUpd/1  "Sync"
  Brake.IF.In/1 -> Brake/2
  VhclCtrl.Brake/1 -> Brake/3
  Sync_In/1 -> Brake/1
  BrakeUpd/2 -> CreateBus Vhcl.Wheel.PT/1(In)
  CreateBus Vhcl.Wheel.PT/1(Out) -> Vhcl.Wheel.PT/1

== system RS_DS_CM11_SimulinkRS/CarMaker/IPG Vehicle/CarAndTrailer ==
  Sync_In : Inport
  VhclCtrl.Steering : Inport  Port=2
  Vhcl.Wheel.In : Inport  Port=3
  Vhcl.Misc : Inport  Port=4
  CarAndTrailerUpd : Subsystem
  Forces : Subsystem
  Ground : Ground
  Kinematics : Subsystem
  Kinetics : Subsystem
  Steering : Subsystem
  Terminator : Terminator
  Terminator1 : Terminator
  Trailer : Subsystem
  Sync_Out : Outport  VectorParamsAs1DForOutWhenUnconnected=off
  Brake.IF.In : Outport  Port=2  VectorParamsAs1DForOutWhenUnconnected=off
  wires:
  Trailer/9(Car.Hitch.FrcTrq) -> CarAndTrailerUpd/9(Car.Hitch.FrcTrq)
  Trailer/8(Vhcl.Wheel.RR) -> CarAndTrailerUpd/8(Vhcl.Wheel.RR)
  Trailer/7(Vhcl.Wheel.RL) -> CarAndTrailerUpd/7(Vhcl.Wheel.RL)
  Trailer/6(Vhcl.Wheel.FR) -> CarAndTrailerUpd/6(Vhcl.Wheel.FR)
  Trailer/5(Vhcl.Wheel.FL) -> CarAndTrailerUpd/5(Vhcl.Wheel.FL)
  Trailer/4(Vhcl.PoI) -> CarAndTrailerUpd/4(Vhcl.PoI)
  Trailer/3(Vhcl.Motion) -> CarAndTrailerUpd/3(Vhcl.Motion)
  Trailer/2(Vhcl.Steering) -> CarAndTrailerUpd/2(Vhcl.Steering)
  Trailer/1(Sync_Out) -> CarAndTrailerUpd/1(Sync_In)
  CarAndTrailerUpd/2(Brake.IF.In) -> Brake.IF.In/1
  CarAndTrailerUpd/1(Sync_Out) -> Sync_Out/1
  Vhcl.Misc/1 -> Terminator1/1
  Vhcl.Wheel.In/1 -> Terminator/1
  Kinetics/6(WheelCarrier.Misc) -> Trailer/6(WheelCarrier.Misc)
  Kinetics/5(Car.Trq_T2W) -> Trailer/5(Car.Trq_T2W)
  Steering/2(Steer.IF) -> Kinematics/2(Steer.IF)
  Kinetics/4(Car.Fr1) -> Trailer/4(Car.Fr1)
  Kinetics/3(Car.Hitch) -> Trailer/3(Car.Hitch)
  Kinetics/2(Trailer.Load) -> Trailer/2(Trailer.Load)
  VhclCtrl.Steering/1 -> Steering/2(VhclCtrl.Steering)
  Sync_In/1 -> Steering/1(Sync_In)
  Steering/1(Sync_Out) -> Kinematics/1(Sync_In)
  Kinetics/1(Sync_Out) -> Trailer/1(Sync_In)
  Ground/1 -> CarAndTrailerUpd/10(Vhcl.Fr1A)
  Forces/11(FStabi_ext) -> Kinetics/11(FStabi_ext)
  Forces/10(FDamp_ext) -> Kinetics/10(FDamp_ext)
  Forces/9(FSpring_ext) -> Kinetics/9(FSpring_ext)
  Forces/8(TireRR_Out) -> Kinetics/8(TireRR.Out)
  Forces/7(TireRL_Out) -> Kinetics/7(TireRL.Out)
  Forces/6(TireFR_Out) -> Kinetics/6(TireFR.Out)
  Forces/5(TireFL_Out) -> Kinetics/5(TireFL.Out)
  Forces/4(Car.Load) -> Kinetics/4(Car.Load)
  Forces/2(Car.Virtual) -> Kinetics/2(Car.Virtual)
  Kinematics/6(lSpring) -> Forces/6(lSpring)
  Kinematics/7(vDamp) -> Forces/7(vDamp)
  Forces/3(Car.Aero) -> Kinetics/3(Car.Aero)
  Forces/1(Sync_Out) -> Kinetics/1(Sync_In)
  Kinematics/5(TireRR_In) -> Forces/5(TireRR_In)
  Kinematics/4(TireRL_In) -> Forces/4(TireRL_In)
  Kinematics/3(TireFR_In) -> Forces/3(TireFR_In)
  Kinematics/2(TireFL_In) -> Forces/2(TireFL_In)
  Kinematics/1(Sync_Out) -> Forces/1(Sync_In)
  Kinematics/8(lStabi) -> Forces/8(lStabi)
  Forces/12(FBuf_ext) -> Kinetics/12(FBuf_ext)
  Kinematics/9(lBuf) -> Forces/9(lBuf)

== system RS_DS_CM11_SimulinkRS/CarMaker/IPG Vehicle/Driver and Drive Cycle ==
  Veh speed feedback [kph] : Inport
  HIL Veh speed Cmd [kph] : Inport  Port=2
  Data Type Conversion11 : DataTypeConversion  OutDataTypeStr=double  LockScale=on
  Driver and PI with FF Control : Subsystem
  Gain : Gain  Gain=1/1.609
  Gain1 : Gain  Gain=1/1.609
  ManSpd : Constant  Value=0
  ManSpdSel : Constant  Value=3
  Multiport Switch1 : MultiPortSwitch
  Rate Limiter : RateLimiter  RisingSlewLimit=5  FallingSlewLimit=-5  SampleTimeMode=inherited
  Terminator : Terminator
  Terminator1 : Terminator
  DriverBus : Outport
  wires:
  [VehSpdKph] -> Data Type Conversion11/1
  Driver and PI with FF Control/1(DriverBus) -> DriverBus/1
  Data Type Conversion11/1 -> Gain/1, Driver and PI with FF Control/1(Vehicle_Spd_kph)  "Vehicle_Spd_kph"
  Gain/1 -> Terminator/1  "Vehicle_Spd_mph"
  Gain1/1 -> Terminator1/1  "Vehicle_SpdDmd_mph"
  Multiport Switch1/1 -> Gain1/1, Driver and PI with FF Control/2(Vehicle_SpdDmd_kph)  "RefSpd [km/hr]"
  ManSpd/1 -> Rate Limiter/1
  Rate Limiter/1 -> Multiport Switch1/2
  ManSpdSel/1 -> Multiport Switch1/1
  [VehSpdKph] -> Multiport Switch1/3
  HIL Veh speed Cmd [kph]/1 -> Multiport Switch1/4
  Veh speed feedback [kph]/1 -> [VehSpdKph]

== system RS_DS_CM11_SimulinkRS/CarMaker/IPG Vehicle/PowerTrain ==
  note: When replacing the entire powertrain,
      | be sure to disable the IPG powertrain model by using the powertrain
      | model 'Model Manager off' in the vehicle GUI.
  note: <Your model here>
  Sync_In : Inport
  Vhcl.Wheel.PT : Inport  Port=2
  VhclCtrl.PT : Inport  Port=3
  BusCreator1 : BusCreator  Inputs=42
  Demux1 : Demux  Outputs=42
      settings: DisplayOption=none
  PowerTrain : S-Function  FunctionName=CM_Sfun  Parameters='PowerTrain'  SFunctionDeploymentMode=off  EnableBusSupport=off
  PowerTrainUpd : S-Function  FunctionName=CM_Sfun  Parameters='PowerTrainUpd'  SFunctionDeploymentMode=off  EnableBusSupport=off
  Sync_Out : Outport  VectorParamsAs1DForOutWhenUnconnected=off
  wires:
  BusCreator1/1 -> PowerTrainUpd/2
  Demux1/42 -> BusCreator1/42  "PT IF WRR Trq_BrakeReg_max"
  Demux1/41 -> BusCreator1/41  "PT IF WRR Trq_BrakeReg"
  Demux1/40 -> BusCreator1/40  "PT IF WRR Trq_Supp2WC"
  Demux1/39 -> BusCreator1/39  "PT IF WRR Trq_Drive"
  Demux1/38 -> BusCreator1/38  "PT IF WRR Trq_B2W"
  Demux1/37 -> BusCreator1/37  "PT IF WRR rotv"
  Demux1/36 -> BusCreator1/36  "PT IF WRR rot"
  Demux1/35 -> BusCreator1/35  "PT IF WRL Trq_BrakeReg_max"
  Demux1/34 -> BusCreator1/34  "PT IF WRL Trq_BrakeReg"
  Demux1/33 -> BusCreator1/33  "PT IF WRL Trq_Supp2WC"
  Demux1/32 -> BusCreator1/32  "PT IF WRL Trq_Drive"
  Demux1/31 -> BusCreator1/31  "PT IF WRL Trq_B2W"
  Demux1/30 -> BusCreator1/30  "PT IF WRL rotv"
  Demux1/29 -> BusCreator1/29  "PT IF WRL rot"
  Demux1/28 -> BusCreator1/28  "PT IF WFR Trq_BrakeReg_max"
  Demux1/27 -> BusCreator1/27  "PT IF WFR Trq_BrakeReg"
  Demux1/26 -> BusCreator1/26  "PT IF WFR Trq_Supp2WC"
  Demux1/25 -> BusCreator1/25  "PT IF WFR Trq_Drive"
  Demux1/24 -> BusCreator1/24  "PT IF WFR Trq_B2W"
  Demux1/23 -> BusCreator1/23  "PT IF WFR rotv"
  Demux1/22 -> BusCreator1/22  "PT IF WFR rot"
  Demux1/21 -> BusCreator1/21  "PT IF WFL Trq_BrakeReg_max"
  Demux1/20 -> BusCreator1/20  "PT IF WFL Trq_BrakeReg"
  Demux1/19 -> BusCreator1/19  "PT IF WFL Trq_Supp2WC"
  Demux1/18 -> BusCreator1/18  "PT IF WFL Trq_Drive"
  Demux1/17 -> BusCreator1/17  "PT IF WFL Trq_B2W"
  Demux1/16 -> BusCreator1/16  "PT IF WFL rotv"
  Demux1/15 -> BusCreator1/15  "PT IF WFL rot"
  Demux1/14 -> BusCreator1/14  "PT IF DL_iDiff_mean"
  Demux1/13 -> BusCreator1/13  "PT IF Trq_Supp2BdyEng y"
  Demux1/12 -> BusCreator1/12  "PT IF Trq_Supp2BdyEng x"
  Demux1/11 -> BusCreator1/11  "PT IF Trq_Supp2Bdy1B z"
  Demux1/10 -> BusCreator1/10  "PT IF Trq_Supp2Bdy1B y"
  Demux1/9 -> BusCreator1/9  "PT IF Trq_Supp2Bdy1B x"
  Demux1/8 -> BusCreator1/8  "PT IF Trq_Supp2Bdy1 z"
  Demux1/7 -> BusCreator1/7  "PT IF Trq_Supp2Bdy1 y"
  Demux1/6 -> BusCreator1/6  "PT IF Trq_Supp2Bdy1 x"
  Demux1/5 -> BusCreator1/5  "PT IF Engine_rotv"
  Demux1/4 -> BusCreator1/4  "PT IF GearNo"
  Demux1/3 -> BusCreator1/3  "PT IF OperationError"
  Demux1/2 -> BusCreator1/2  "PT IF OperationState"
  Demux1/1 -> BusCreator1/1  "PT IF Ignition"
  Sync_In/1 -> PowerTrain/1
  PowerTrain/2 -> Demux1/1
  PowerTrainUpd/1 -> Sync_Out/1
  PowerTrain/1 -> PowerTrainUpd/1  "Sync"
  VhclCtrl.PT/1 -> PowerTrain/3
  Vhcl.Wheel.PT/1 -> PowerTrain/2

== system RS_DS_CM11_SimulinkRS/CarMaker/RealSim Core/dSPACE TCP In ==
  Data Type Conversion1 : DataTypeConversion  OutDataTypeStr=uint8
  Data Type Conversion4 : DataTypeConversion  OutDataTypeStr=double
  Display7 : Display
  Ethernet Setup (1) : dsmpblib/Data Inport  Priority=10000
      settings: SourceProductName=dSPACE Model Interface Blockset
  Receive_In [TCP (1)] : dsmpblib/Data Inport  Priority=10000
      settings: SourceProductName=dSPACE Model Interface Blockset
  Receive_Out [TCP (1)] : dsmpblib/Data Outport  Priority=-10000
      settings: SourceProductName=dSPACE Model Interface Blockset
  Status/Control_In [TCP (1)] : dsmpblib/Data Inport  Priority=10000
      settings: SourceProductName=dSPACE Model Interface Blockset
  Terminator{19,25..27} (4 alike) : Terminator
  Transmit_In [TCP (1)] : dsmpblib/Data Inport  Priority=10000
      settings: SourceProductName=dSPACE Model Interface Blockset
  ByteData : Outport
  nByte : Outport  Port=2
  ConnectionState : Outport  Port=3
  wires:
  Data Type Conversion4/1 -> ConnectionState/1  "ConnectionState"
  Status/Control_In [TCP (1)]/1 -> Data Type Conversion4/1  "Connection_State"
  Receive_In [TCP (1)]/4 -> Receive_Out [TCP (1)]/1
  Ethernet Setup (1)/1 -> Terminator26/1
  Receive_In [TCP (1)]/1 -> Data Type Conversion1/1
  Transmit_In [TCP (1)]/2 -> Terminator19/1
  Transmit_In [TCP (1)]/1 -> Terminator27/1
  Receive_In [TCP (1)]/2 -> Terminator25/1
  Receive_In [TCP (1)]/3 -> Display7/1, nByte/1
  Data Type Conversion1/1 -> ByteData/1

== system RS_DS_CM11_SimulinkRS/CarMaker/RealSim Core/dSPACE TCP Out ==
  ByteSend : Inport
  nMsgSend : Inport  Port=2
  sendTrigger : Inport  Port=3
  Constant1 : Constant  Value=0
  Data Type Conversion4 : DataTypeConversion
  Display7 : Display
  Transmit_Out [TCP (1)] : dsmpblib/Data Outport  Priority=-10000
      settings: SourceProductName=dSPACE Model Interface Blockset
  switch for 0.1 send out : Switch  Criteria=u2 > Threshold
  wires:
  Constant1/1 -> switch for 0.1 send out/3
  nMsgSend/1 -> Data Type Conversion4/1
  Data Type Conversion4/1 -> switch for 0.1 send out/1, Display7/1
  switch for 0.1 send out/1 -> Transmit_Out [TCP (1)]/2  "sendByteSize_RealSimPack"
  ByteSend/1 -> Transmit_Out [TCP (1)]/1
  sendTrigger/1 -> switch for 0.1 send out/2

== system RS_DS_CM11_SimulinkRS/CarMaker/RealSim Translate CM Signal to Bus as Feedback to SUMO//VISSIM/RealSim CreatBus ==
  note: activeLaneChange is set more for VISSIM co-simulation
  In : Inport
  positionX : Inport  Port=2
  positionY : Inport  Port=3
  positionZ : Inport  Port=4
  heading : Inport  Port=5
  color : Inport  Port=6
  speedDesired : Inport  Port=7
  Bus Creator1 : BusCreator  Inputs=36  OutDataTypeStr=Bus: VehDataBus
  Bus Selector1 : BusSelector  OutputSignals=id,idLength,type,typeLength,vehicleClass,vehicleClassLength,speed,acceleration,positionX,positionY,positionZ,heading,color,linkId,linkIdLength,laneId,distanceTravel,speedDesired,accelerationDesired,hasPrecedingVehicle,precedingVehicleId,precedingVehicleIdLength,precedingVehicleDistance,precedingVehicleSpeed,signalLightId,signalLightIdLength,signalLightHeadId,signalLightDistance,signalLightColor,speedLimit,speedLimitNext,speedLimitChangeDistance,linkIdNext,linkIdNextLength,grade,activeLaneChange
  Terminator{,1..6} (7 alike) : Terminator
  activeLaneChange : Constant  Value=0
  Out : Outport
  wires:
  Bus Selector1/1 -> Bus Creator1/1  "<id>"
  Bus Selector1/2 -> Bus Creator1/2  "<idLength>"
  Bus Selector1/3 -> Bus Creator1/3  "<type>"
  Bus Selector1/4 -> Bus Creator1/4  "<typeLength>"
  Bus Selector1/5 -> Bus Creator1/5  "<vehicleClass>"
  Bus Selector1/6 -> Bus Creator1/6  "<vehicleClassLength>"
  Bus Selector1/7 -> Bus Creator1/7  "<speed>"
  Bus Selector1/8 -> Bus Creator1/8  "<acceleration>"
  Bus Selector1/9 -> Terminator6/1  "<positionX>"
  Bus Selector1/10 -> Terminator5/1  "<positionY>"
  Bus Selector1/11 -> Terminator4/1  "<positionZ>"
  Bus Selector1/12 -> Terminator1/1  "<heading>"
  Bus Selector1/13 -> Terminator3/1  "<color>"
  Bus Selector1/14 -> Bus Creator1/14  "<linkId>"
  Bus Selector1/15 -> Bus Creator1/15  "<linkIdLength>"
  Bus Selector1/16 -> Bus Creator1/16  "<laneId>"
  Bus Selector1/17 -> Bus Creator1/17  "<distanceTravel>"
  Bus Selector1/18 -> Terminator2/1  "<speedDesired>"
  Bus Selector1/19 -> Bus Creator1/19  "<accelerationDesired>"
  Bus Selector1/20 -> Bus Creator1/20  "<hasPrecedingVehicle>"
  Bus Selector1/21 -> Bus Creator1/21  "<precedingVehicleId>"
  Bus Selector1/22 -> Bus Creator1/22  "<precedingVehicleIdLength>"
  Bus Selector1/23 -> Bus Creator1/23  "<precedingVehicleDistance>"
  Bus Selector1/24 -> Bus Creator1/24  "<precedingVehicleSpeed>"
  Bus Selector1/25 -> Bus Creator1/25  "<signalLightId>"
  Bus Selector1/26 -> Bus Creator1/26  "<signalLightIdLength>"
  Bus Selector1/27 -> Bus Creator1/27  "<signalLightHeadId>"
  Bus Selector1/28 -> Bus Creator1/28  "<signalLightDistance>"
  Bus Selector1/29 -> Bus Creator1/29  "<signalLightColor>"
  Bus Selector1/30 -> Bus Creator1/30  "<speedLimit>"
  Bus Selector1/31 -> Bus Creator1/31  "<speedLimitNext>"
  Bus Selector1/32 -> Bus Creator1/32  "<speedLimitChangeDistance>"
  Bus Selector1/33 -> Bus Creator1/33  "<linkIdNext>"
  Bus Selector1/34 -> Bus Creator1/34  "<linkIdNextLength>"
  Bus Selector1/36 -> Terminator/1  "<activeLaneChange>"
  positionY/1 -> Bus Creator1/10  "positionY"
  heading/1 -> Bus Creator1/12  "heading"
  color/1 -> Bus Creator1/13  "color"
  positionX/1 -> Bus Creator1/9  "positionX"
  speedDesired/1 -> Bus Creator1/18  "speedDesired"
  positionZ/1 -> Bus Creator1/11  "positionZ"
  Bus Creator1/1 -> Out/1
  In/1 -> Bus Selector1/1
  activeLaneChange/1 -> Bus Creator1/36  "activeLaneChange"
  Bus Selector1/35 -> Bus Creator1/35  "<grade>"
